simulink library "controller_library"  (R2016b)
settings: Solver=VariableStepAuto  StartTime=0.0  StopTime=10.0  RelTol=1e-3
undefined symbols (not defined in the file or in its folder): ControlParams
settings Model: Creator=gyk  LastModifiedBy=gyk

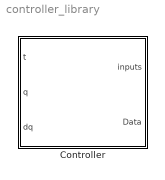
== system controller_library ==
  Controller : Subsystem

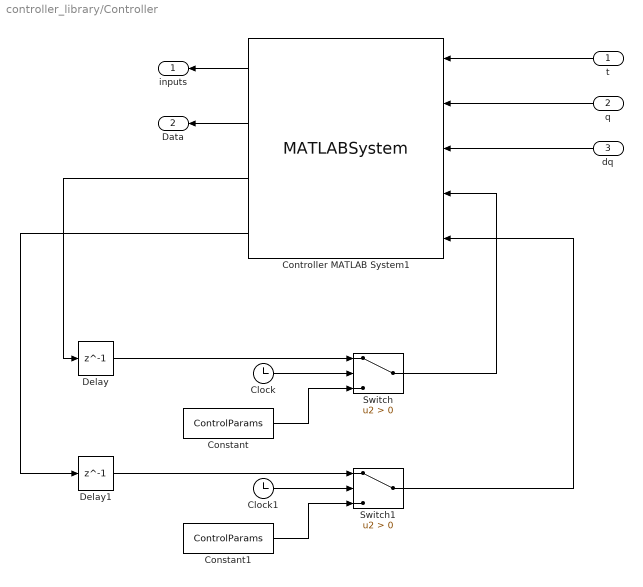
== system controller_library/Controller ==
  t : Inport
  q : Inport  Port=2
  dq : Inport  Port=3
  Clock : Clock
  Clock1 : Clock
  Constant : Constant  Value=ControlParams  OutDataTypeStr=Bus: cassieControlParamsBus
  Constant1 : Constant  Value=ControlParams  OutDataTypeStr=Bus: cassieControlParamsBus
  Controller MATLAB System1 : MATLABSystem  System=controller.Controller  SimulateUsing=Code generation
      mask Type: controller.Controller
      mask Display:
      | disp('Controller');
      | port_label('input',1,'t');
      | port_label('input',2,'q');
      | port_label('input',3,'dq');
      | port_label('input',4,'params');
      | port_label('input',5,'states');
      | port_label('output',1,'inputs');
      | port_label('output',2,'Data');
      | port_label('output',3,'params');
      | port_label('output',4,'states');
  Delay : Delay  DelayLength=1  InitialCondition=0
  Delay1 : Delay  DelayLength=1  InitialCondition=0
  Switch : Switch  Criteria=u2 > Threshold
  Switch1 : Switch  Criteria=u2 > Threshold
  inputs : Outport
  Data : Outport  Port=2
  wires:
  t/1 -> Controller MATLAB System1/1
  dq/1 -> Controller MATLAB System1/3
  q/1 -> Controller MATLAB System1/2
  Controller MATLAB System1/1 -> inputs/1
  Constant/1 -> Switch/3
  Controller MATLAB System1/3 -> Delay/1
  Delay/1 -> Switch/1
  Clock/1 -> Switch/2
  Constant1/1 -> Switch1/3
  Delay1/1 -> Switch1/1
  Clock1/1 -> Switch1/2
  Controller MATLAB System1/4 -> Delay1/1
  Switch/1 -> Controller MATLAB System1/4
  Switch1/1 -> Controller MATLAB System1/5
  Controller MATLAB System1/2 -> Data/1
